simulink model "Ball_bounce"  (R2014a)
settings: Solver=ode45  StartTime=0.0  StopTime=20  FixedStep=0.1  MaxStep=0.01  RelTol=1e-3  AbsTol=1E-6
libraries: simulink x1
Description:
  | Bouncing Ball Model
  | 
  | This model calculates the trajectory, over time, of a ball thrown
  | upward with a velocity of 15 meters per second from a height of 10 m.
  | The model demonstrates the use of the 'ReinitDXDTwhenXreachesSaturation'
  | parameter in the Second-Order Integrator block to model this system.
  | This parameter, when set to 'on', forces a reinitialization of dx/dt
  | (velocity in the model) at the instant when x (position) reaches
  | saturation (i.e., when the ball hits the ground). The reinitialized value
  | is calculated by multiplying a coefficient of restitution times the ball
  | velocity, the instant before the ball hits the ground. The Memory block
  | in the calculation loop serves to capture the velocity of the ball just
  | before it hits the ground. The position of the ball is plotted in the
  | upper axis of the scope while the velocity of the ball is plotted in
  | the lower axis.
settings Model: Creator=The MathWorks Inc.  LastModifiedBy=李广文
settings DataIOCC: LimitDataPoints=off  MaxDataPoints=7500  SaveOutput=off  SignalLogging=off  DSMLogging=off  SaveTime=off
settings OptimizationCC: ExpressionDepthLimit=2147483647  EfficientFloat2IntCast=on
settings DebuggingCC: UnderspecifiedInitializationDetection=Classic  IgnoredZcDiagnostic=none  SolverPrmCheckMsg=none  FcnCallInpInsideContextMsg=EnableAllAsWarning  StateNameClashWarn=warning
settings HardwareCC: TargetLongLongMode=on  TargetEndianess=LittleEndian  TargetHWDeviceType=MATLAB Host  ProdEqTarget=off
settings RTWCC: SystemTargetFile=rsim.tlc  TemplateMakefile=rsim_default_tmf  Description=Rapid Simulation Target  ProcessScript=rsim_make_rtw_hook
settings RSimTargetCC: ERTMultiwordTypeDef=System defined  ERTMultiwordLength=256  EnableShiftOperators=on

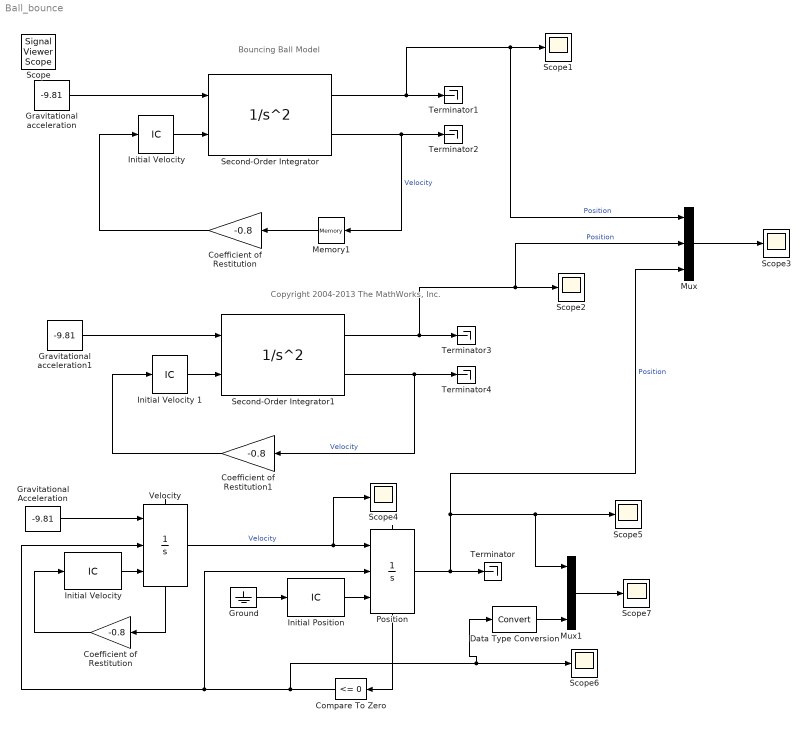
== system Ball_bounce ==
  note: Copyright 2004-2013 The MathWorks, Inc.
  note: Bouncing Ball Model
  Coefficient of Restitution : Gain  Gain=-0.8
  Coefficient of Restitution1 : Gain  Gain=-0.8
  Coefficient of Restitution : Gain  Gain=-0.8  SaturateOnIntegerOverflow=on  OutDataTypeStr=Inherit: Same as input  ParamDataTypeStr=Inherit: Same as input
  Compare To Zero : simulink/Logic and Bit Operations/Compare To Zero  relop=<=  OutDataTypeStr=boolean
  Data Type Conversion : DataTypeConversion
  Gravitational Acceleration : Constant  Value=-9.81
  Gravitational acceleration : Constant  Value=-9.81  OutDataTypeStr=double
  Gravitational acceleration1 : Constant  Value=-9.81  OutDataTypeStr=double
  Ground : Ground
  "Initial Velocity " : InitialCondition  Value=15
  Initial Velocity 1 : InitialCondition  Value=15
  Initial Position : InitialCondition  Value=10
  Initial Velocity : InitialCondition  Value=15
  Memory1 : Memory
  Mux : Mux  Inputs=3
  Mux1 : Mux  Inputs=3
  Position : Integrator  ExternalReset=rising  InitialConditionSource=external  LimitOutput=on  LowerSaturationLimit=0  ShowStatePort=on
  Scope{1..7} (7 alike) : Scope
      Scope3 settings: SaveName=ScopeData2
      Scope4 settings: SaveName=ScopeData3
      Scope5 settings: SaveName=ScopeData4
      Scope6 settings: SaveName=ScopeData5
      Scope7 settings: SaveName=ScopeData6
  Second-Order Integrator : SecondOrderIntegrator  ICX=10.0  LimitX=on  LowerLimitX=0  StateNameX='Position'  ICSourceDXDT=external  StateNameDXDT='Velocity'  ReinitDXDTwhenXreachesSaturation=on
  Second-Order Integrator1 : SecondOrderIntegrator  ICX=10.0  LimitX=on  LowerLimitX=0  StateNameX='Position'  ICSourceDXDT=external  StateNameDXDT='Velocity'  ReinitDXDTwhenXreachesSaturation=on
  Terminator{,1..4} (5 alike) : Terminator
  Velocity : Integrator  ExternalReset=rising  InitialConditionSource=external  ShowStatePort=on
  Scope : SignalViewerScope  IOType=viewer  NumInputPorts=2  RefreshTime=0.035000
      settings: TimeRange=25  YMin=0~-30  YMax=25~20
  wires:
  Gravitational acceleration/1 -> Second-Order Integrator/1
  Second-Order Integrator/1 -> Mux/1, Scope1/1, Terminator1/1  "Position"
  Second-Order Integrator/2 -> Memory1/1, Terminator2/1  "Velocity"
  "Initial Velocity "/1 -> Second-Order Integrator/2
  Coefficient of Restitution/1 -> "Initial Velocity "/1
  Memory1/1 -> Coefficient of Restitution/1
  Gravitational acceleration1/1 -> Second-Order Integrator1/1
  Second-Order Integrator1/1 -> Terminator3/1, Mux/2, Scope2/1  "Position"
  Second-Order Integrator1/2 -> Coefficient of Restitution1/1, Terminator4/1  "Velocity"
  Initial Velocity 1/1 -> Second-Order Integrator1/2
  Coefficient of Restitution1/1 -> Initial Velocity 1/1
  Mux/1 -> Scope3/1
  Initial Velocity/1 -> Velocity/3
  Coefficient of Restitution/1 -> Initial Velocity/1
  Velocity/1 -> Scope4/1, Position/1  "Velocity"
  Gravitational Acceleration/1 -> Velocity/1
  Ground/1 -> Initial Position/1
  Compare To Zero/1 -> Data Type Conversion/1, Scope6/1, Velocity/2, Position/2
  Initial Position/1 -> Position/3
  Position/1 -> Mux1/1, Scope5/1, Mux/3, Terminator/1  "Position"
  Position/State -> Compare To Zero/1
  Velocity/State -> Coefficient of Restitution/1
  Mux1/1 -> Scope7/1
  Data Type Conversion/1 -> Mux1/3
